simulink model "FrequencyTestModel"  (R2021a)
settings: Solver=FixedStepAuto  StartTime=0.0  StopTime=2  FixedStep=0.001  RelTol=1e-3
settings Model: Creator=Mertcan  LastModifiedBy=Mertcan

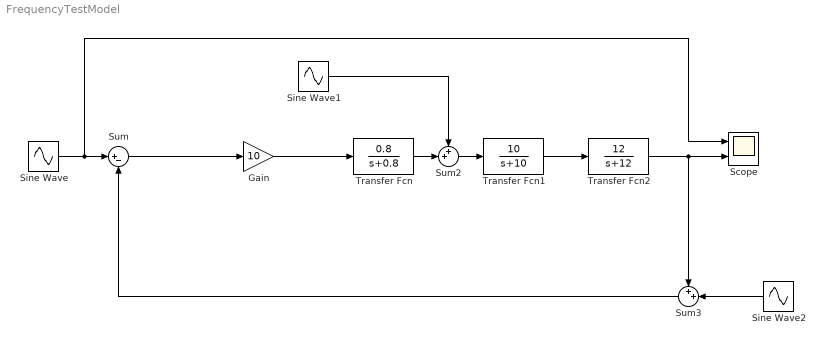
== system FrequencyTestModel ==
  Gain : Gain  Gain=10
  Scope : Scope  NumInputPorts=2
  Sine Wave : Sin  Frequency=20  SampleTime=0
  Sine Wave1 : Sin  Amplitude=0  Frequency=2*pi*0.1  SampleTime=0
  Sine Wave2 : Sin  Amplitude=0  Frequency=2*pi*20  SampleTime=0
  Sum : Sum  Inputs=|+-
  Sum2 : Sum  Inputs=++|
  Sum3 : Sum  Inputs=++|
  Transfer Fcn : TransferFcn  Numerator=[0.8]  Denominator=[1 0.8]
  Transfer Fcn1 : TransferFcn  Numerator=[10]  Denominator=[1 10]
  Transfer Fcn2 : TransferFcn  Numerator=[12]  Denominator=[1 12]
  wires:
  Transfer Fcn/1 -> Sum2/2
  Sum2/1 -> Transfer Fcn1/1
  Transfer Fcn1/1 -> Transfer Fcn2/1
  Sum3/1 -> Sum/2
  Transfer Fcn2/1 -> Scope/2, Sum3/1
  Sine Wave/1 -> Scope/1, Sum/1
  Sine Wave1/1 -> Sum2/1
  Gain/1 -> Transfer Fcn/1
  Sum/1 -> Gain/1
  Sine Wave2/1 -> Sum3/2
